simulink model "Tavola3_tretras_FL"  (R2018b)
settings: Solver=FixedStepAuto  StartTime=0.0  StopTime=80  RelTol=1e-3
undefined symbols (not defined in the file or in its folder): sigbuilder_block
libraries: simulink x1
settings Model: Creator=Utente  LastModifiedBy=Utente

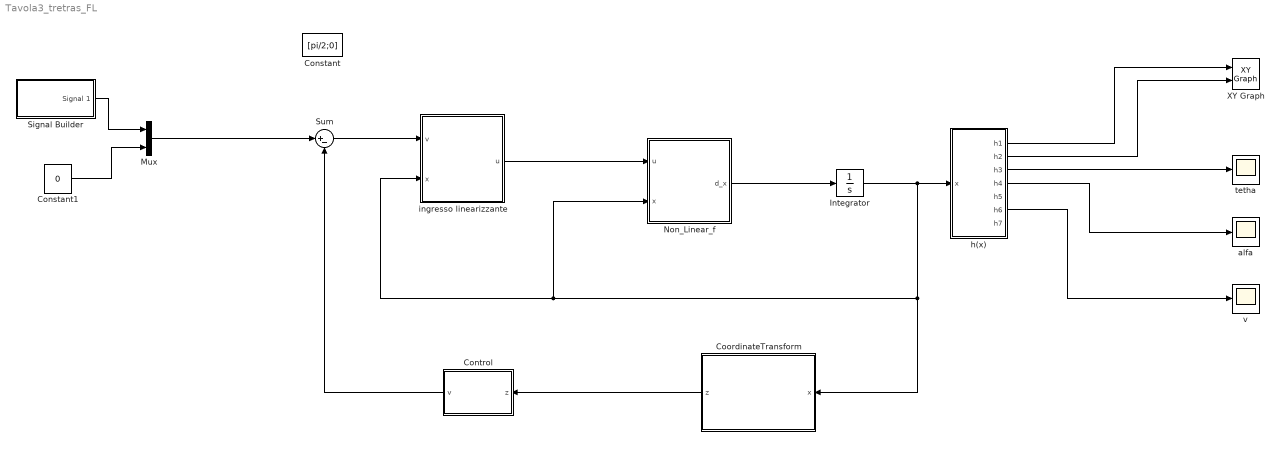
== system Tavola3_tretras_FL ==
  Constant : Constant  Value=[pi/2;0]
  Constant1 : Constant  Value=0
  Control : MATLAB Function  TreatAsAtomicUnit=on
  CoordinateTransform : MATLAB Function  TreatAsAtomicUnit=on
  Integrator : Integrator  InitialCondition=[0,0,0,0.17,0,5,0]
  Mux : Mux  Inputs=2
  "Non_Linear_f " : MATLAB Function  TreatAsAtomicUnit=on
  Signal Builder : Subsystem  Tag=STV Subsys  LoadFcn=sigbuilder_block('load');  StartFcn=sigbuilder_block('start');  StopFcn=sigbuilder_block('stop');  ClipboardFcn=sigbuilder_block('clipboard');  mask(Sigbuilder block){tuvar=[0:10]}
      mask help: Simulink:masks:SigbuilderBlock_MD
      mask init:
      | if ~strcmp(get_param(bdroot(gcbh),'SimulationStatus'),'stopped') tuvar = sigbuilder_block('maskInit'); end
      settings: CopyFcn=sigbuilder_block('copy');  DeleteFcn=sigbuilder_block('delete');  ModelCloseFcn=sigbuilder_block('modelClose');  PreSaveFcn=sigbuilder_block('preSave');  PauseFcn=sigbuilder_block('pause');  ContinueFcn=sigbuilder_block('continue');  NameChangeFcn=sigbuilder_block('namechange');  OpenFcn=sigbuilder_block('open',[437.6 199.2 731.65 400 ]);  CloseFcn=sigbuilder_block('close');
      mask Display: plot(0, 0, 100, 100,[2, 2, 32, 32, 2], [68, 8, 8, 68, 68],[32, 2], [38, 38], [32, 19, 2],[53, 60, 44], [32, 17, 17, 2],[16, 16, 31, 31]);txt = getActiveGroup(gcbh);text(2, 100, txt,'verticalAlignment', 'top');
  Sum : Sum  Inputs=|+-
  XY Graph : simulink/Sinks/XY Graph  xmin=-100  xmax=100  ymin=-100  ymax=100  st=-1
  alfa : Scope
  h(x) : MATLAB Function  TreatAsAtomicUnit=on
  ingresso linearizzante : MATLAB Function  TreatAsAtomicUnit=on
  tetha : Scope
  v : Scope
  wires:
  "Non_Linear_f "/1(d_x) -> Integrator/1
  Integrator/1 -> "Non_Linear_f "/2(x), ingresso linearizzante/2(x), CoordinateTransform/1(x), h(x)/1(x)
  ingresso linearizzante/1(u) -> "Non_Linear_f "/1(u)
  Sum/1 -> ingresso linearizzante/1(v)
  h(x)/3(h3) -> tetha/1
  h(x)/4(h4) -> alfa/1
  CoordinateTransform/1(z) -> Control/1(z)
  h(x)/1(h1) -> XY Graph/1
  h(x)/2(h2) -> XY Graph/2
  h(x)/6(h6) -> v/1
  Control/1(v) -> Sum/2
  Constant1/1 -> Mux/2
  Mux/1 -> Sum/1
  Signal Builder/1(Signal 1) -> Mux/1

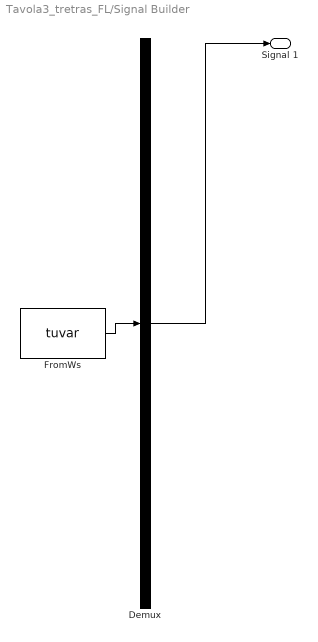
== system Tavola3_tretras_FL/Signal Builder ==
  Demux : Demux  Tag=STV Demux  Outputs=1
  FromWs : FromWorkspace  Tag=STV FromWs  VariableName=tuvar  SampleTime=0
      SigBuilderData=|
      | common.afterFinalStr = 'Extrapolate'
      | common.sampleTime = 0
      | dataSet.timeRange = [0 100]
      | dataSet.name = 'Group 1'
      | sbobj.Groups.Name = 'Group 1'
      | sbobj.Groups.Signals.Name = 'Signal 1'
      | sbobj.Groups.Signals.XData = [0 0.9 50 50 100]
      | sbobj.Groups.Signals.YData = [0 0 6.28 0 6.28]
      | sbobj.Groups.TimeRange = [0 100]
  Signal 1 : Outport  Tag=STV Outport
  wires:
  Demux/1 -> Signal 1/1
  FromWs/1 -> Demux/1

== matlab function Tavola3_tretras_FL/h(x) ==
  data: x input; h1 output; h2 output; h3 output; h4 output; h5 output; h6 output; h7 output
function [h1,h2,h3,h4,h5,h6,h7] = h(x)

x1 = x(1);
x2 = x(2);
x3 = x(3);
x4 = x(4);
x5 = x(5);
x6 = x(6);
x7 = x(7);


h1 = x1;
h2 = x2;
h3 = x3;
h4 = x4;
h5 = x5;
h6 = x6;
h7 = x7;

== matlab function Tavola3_tretras_FL/Non_Linear_f  ==
  data: u input; d_x output; x input
function d_x = statespacef(u,x)

x1 = x(1);
x2 = x(2);
x3 = x(3);
x4 = x(4);
x5 = x(5);
x6 = x(6);
x7 = x(7);


f =                                                                                                                               [x6*cos(x3);
                                                                                                                                  x6*sin(x3);
                                                                                                                                          x7;
                                                                                                                                          x5;
 (2.39*sin(2.0*x4)*x5^2)/(4.79*cos(x4)^2 - 12.5) - (173.0*sin(x4))/(4.79*cos(x4)^2 - 12.5) - (3.28*x7^2*sin(2.0*x4))/(4.79*cos(x4)^2 - 12.5);
       (1.99*sin(3.0*x4) - 6.77*sin(x4))*x7^2 + (23.5*sin(2.0*x4))/(4.79*cos(x4)^2 - 12.5) - (2.19*x5^2*sin(2.0*x4))/(4.79*cos(x4)^2 - 12.5);
                                       (0.547*x6*x7*sin(x4))/(0.228*cos(x4)^2 - 0.315) + (0.228*x5*x7*sin(2.0*x4))/(0.228*cos(x4)^2 - 0.315)];
g1 = [                                              0;
                                                    0;
                                                    0;
                                                    0;
        (2.19*cos(x3) + 3.11)/(4.79*cos(x4)^2 - 12.5);
 -(1.0*(0.547*cos(x4) + 1.0))/(4.79*cos(x4)^2 - 12.5);
                      -0.05/(0.228*cos(x4)^2 - 0.315);];
 
g2 = [                                              0;
                                                    0;
                                                    0;
                                                    0;
        (2.19*cos(x3) + 3.11)/(4.79*cos(x4)^2 - 12.5);
 -(1.0*(0.547*cos(x4) + 1.0))/(4.79*cos(x4)^2 - 12.5);
                       0.05/(0.228*cos(x4)^2 - 0.315)];
d_x = f + [g1,g2]*u;

== matlab function Tavola3_tretras_FL/ingresso linearizzante ==
  data: v input; u output; x input
function u = inputLinearizzante(v,x)

x1 = x(1);
x2 = x(2);
x3 = x(3);
x4 = x(4);
x5 = x(5);
x6 = x(6);
x7 = x(7);

inv_E =  [ 3.15 - 2.28*cos(x4)^2, (18.1*(33.0*cos(x4)^2 - 86.0))/(547.0*cos(x3) + 778.0);
           2.28*cos(x4)^2 - 3.15, (18.1*(33.0*cos(x4)^2 - 86.0))/(547.0*cos(x3) + 778.0)];
       
Gamma =                                [(0.547*x6*x7*sin(x4))/(0.228*cos(x4)^2 - 0.315) + (0.228*x5*x7*sin(2.0*x4))/(0.228*cos(x4)^2 - 0.315);
 (2.39*sin(2.0*x4)*x5^2)/(4.79*cos(x4)^2 - 12.5) - (173.0*sin(x4))/(4.79*cos(x4)^2 - 12.5) - (3.28*x7^2*sin(2.0*x4))/(4.79*cos(x4)^2 - 12.5)];



u = -inv_E*Gamma+inv_E*v;

== matlab function Tavola3_tretras_FL/CoordinateTransform ==
  data: z output; x input
function z = transformCoordinate(x)

x1 = x(1);
x2 = x(2);
x3 = x(3);
x4 = x(4);
x5 = x(5);
x6 = x(6);
x7 = x(7);

                                        z =  [                                                         x3;
                                                                                                       x7;
                                                                                                       x4;
                                                                                                       x5;
                                                                                                       x1;
                                                                                                       x2;
 (x5*(0.547*cos(x4) + 1.0))/(4.79*cos(x4)^2 - 12.5) + (x6*(2.19*cos(x3) + 3.11))/(4.79*cos(x4)^2 - 12.5);];

== matlab function Tavola3_tretras_FL/Control ==
  data: v output; z input
function v = control(z)

    z1 = z(1);
    z2 = z(2);
    z3 = z(3);
    z4 = z(4);
    z5 = z(5);
    z6 = z(6);
    z7 = z(7);

    k11 = 1;
    k12 = 1;
    k21 = 50;
    k22 = 1000;

%     PD
    v1 = k11*z1+k12*z2;
    v2 = k21*z3+k22*z4;
    % v1 = k11*z5;
    % v2 = k21*z6;

    v = [v1;v2];

end
